simulink model "BrainihacksSampleDesignFinal"  (R2021b)
settings: Solver=VariableStepAuto  StartTime=0.0  StopTime=inf  RelTol=1e-3
undefined symbols (not defined in the file): fdesignblkfcn, gcbh, UN
libraries: dsparch4 x6, dspstat3 x2, simulink x2, slrealtimeiplib x1, UnicornLib x1
settings Model: Creator=Jos  LastModifiedBy=Jos

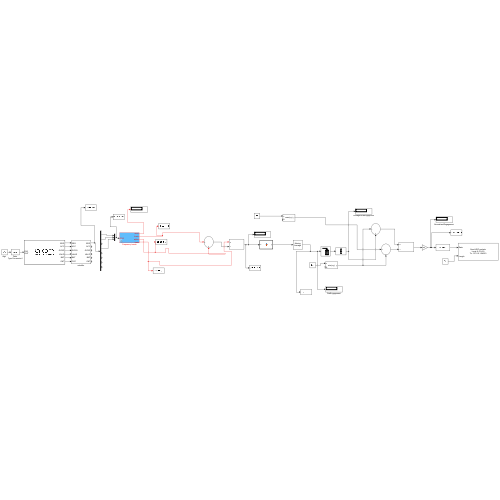
[thumbnail: Simulink's stored preview of the top-level diagram]
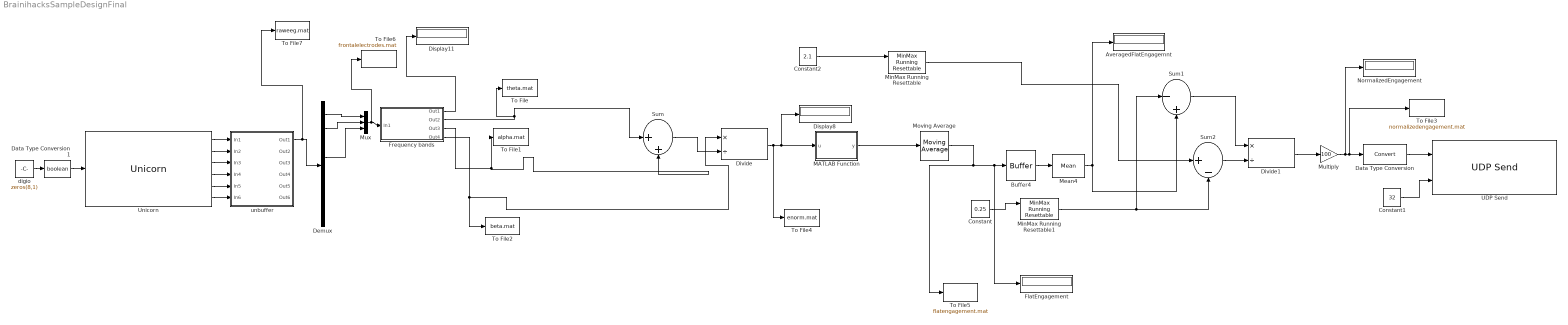
== system BrainihacksSampleDesignFinal ==
  AveragedFlatEngagemnt : Display
  Buffer4 : Buffer  N=128  OutputFrames=off
  Constant : Constant  Value=0.25
  Constant1 : Constant  Value=32
  Constant2 : Constant  Value=2.1
  Data Type Conversion1 : DataTypeConversion  OutDataTypeStr=boolean
  Data Type Conversion : DataTypeConversion
  Demux : Demux  Outputs=8
  Display11 : Display
  Display8 : Display
  Divide : Product  Inputs=*/
  Divide1 : Product  Inputs=*/
  FlatEngagement : Display
  Frequency bands : Subsystem  mask{windowLength=250, windowOverlap=240}
      mask prompts: windowLength "Window Length:"; windowOverlap "Window Overlap:"
      mask Display:
      | port_label('input',1,'EEG')
      | port_label('output',1,'delta')
      | port_label('output',2,'theta')
      | port_label('output',3,'alpha')
      | port_label('output',4,'beta')
  MATLAB Function : MATLAB Function  TreatAsAtomicUnit=on
  Mean4 : dspstat3/Mean  run=off  InputProcessing=Columns as channels (frame based)  reset_popup=None  directionMode=Each column  dimension=1  roiEnable=off  roiType=Rectangles  roiPortion=Entire ROI  roiOutput=Individual statistics for each ROI  roiFlag=off  roundingMode=Floor  overflowMode=off  outputDataTypeStr=Inherit: Same as accumulator  outputMin=[]  outputMax=[]  outputLastDataTypeStr=Inherit: Same as accumulator
  MinMax Running Resettable : simulink/Math Operations/MinMax Running Resettable  Function=max  vinit=0.0
  MinMax Running Resettable1 : simulink/Math Operations/MinMax Running Resettable  Function=min  vinit=0.0
  Moving Average : dspstat3/Moving Average  Method=Exponential weighting  ForgettingFactorPort=off  SpecifyWindowLength=on  WindowLength=4  ForgettingFactor=0.9  SimulateUsing=Code generation
  Multiply : Gain  Gain=100
  Mux : Mux  Inputs=3
  NormalizedEngagement : Display
  Sum : Sum  Inputs=|++
  Sum1 : Sum  Inputs=|-+
  Sum2 : Sum  Inputs=|+-
  To File : ToFile  Filename=theta.mat  SaveFormat=Timeseries
  To File1 : ToFile  Filename=alpha.mat  SaveFormat=Timeseries
  To File2 : ToFile  Filename=beta.mat  SaveFormat=Timeseries
  To File3 : ToFile  Filename=normalizedengagement.mat  SaveFormat=Timeseries
  To File4 : ToFile  Filename=enorm.mat  SaveFormat=Timeseries
  To File5 : ToFile  Filename=flatengagement.mat  SaveFormat=Timeseries
  To File6 : ToFile  Filename=frontalelectrodes.mat  SaveFormat=Timeseries
  To File7 : ToFile  Filename=raweeg.mat  SaveFormat=Timeseries
  UDP Send : slrealtimeiplib/UDP Send  useHostTargetConn=off  toAddress='127.0.0.1'  toPort=54320  sampleTime=-1
      settings: SourceProductBaseCode=XP
  Unicorn : UnicornLib/Unicorn  serial=UN-2019.05.55  old_serial=UN-2019.05.55  frame_length=1  input_source=Electrode
      settings: SourceProductName=Unicorn
  digio : Constant  Value=zeros(8,1)  SampleTime=-1
  "unbuffer " : Subsystem
      mask Display:
      | port_label('input',1,'EEG')
      | port_label('input',2,'ACC')
      | port_label('input',3,'GYRO')
      | port_label('input',4,'VALID')
      | port_label('input',5,'BAT')
      | port_label('input',6,'CNT')
      | port_label('output',1,'EEG')
      | port_label('output',2,'ACC')
      | port_label('output',3,'GYRO')
      | port_label('output',4,'VALID')
      | port_label('output',5,'BAT')
      | port_label('output',6,'CNT')
  wires:
  Unicorn/2 -> "unbuffer "/2(In2)
  Data Type Conversion1/1 -> Unicorn/1
  Unicorn/4 -> "unbuffer "/4(In4)
  Unicorn/5 -> "unbuffer "/5(In5)
  digio/1 -> Data Type Conversion1/1
  Unicorn/3 -> "unbuffer "/3(In3)
  Unicorn/6 -> "unbuffer "/6(In6)
  Unicorn/1 -> "unbuffer "/1(In1)
  Sum1/1 -> Divide1/1
  MinMax Running Resettable1/1 -> Sum1/1, Sum2/2
  Frequency bands/3(Out3) -> Sum/2, To File1/1
  Constant1/1 -> UDP Send/2
  Sum2/1 -> Divide1/2
  Sum/1 -> Divide/2
  MinMax Running Resettable/1 -> Sum2/1
  Data Type Conversion/1 -> UDP Send/1
  Frequency bands/4(Out4) -> Divide/1, To File2/1
  Constant/1 -> MinMax Running Resettable1/1
  Multiply/1 -> NormalizedEngagement/1, To File3/1, Data Type Conversion/1
  "unbuffer "/1(Out1) -> To File7/1, Demux/1
  Mux/1 -> To File6/1, Frequency bands/1(In1)
  Demux/1 -> Mux/1
  Demux/2 -> Mux/2
  Demux/4 -> Mux/3
  Divide1/1 -> Multiply/1
  Frequency bands/2(Out2) -> Sum/1, To File/1
  Buffer4/1 -> Mean4/1
  Mean4/1 -> Sum1/2, AveragedFlatEngagemnt/1
  Constant2/1 -> MinMax Running Resettable/1
  Moving Average/1 -> Buffer4/1, FlatEngagement/1, To File5/1
  Divide/1 -> Display8/1, MATLAB Function/1(u), To File4/1
  MATLAB Function/1(y) -> Moving Average/1
  Frequency bands/1(Out1) -> Display11/1

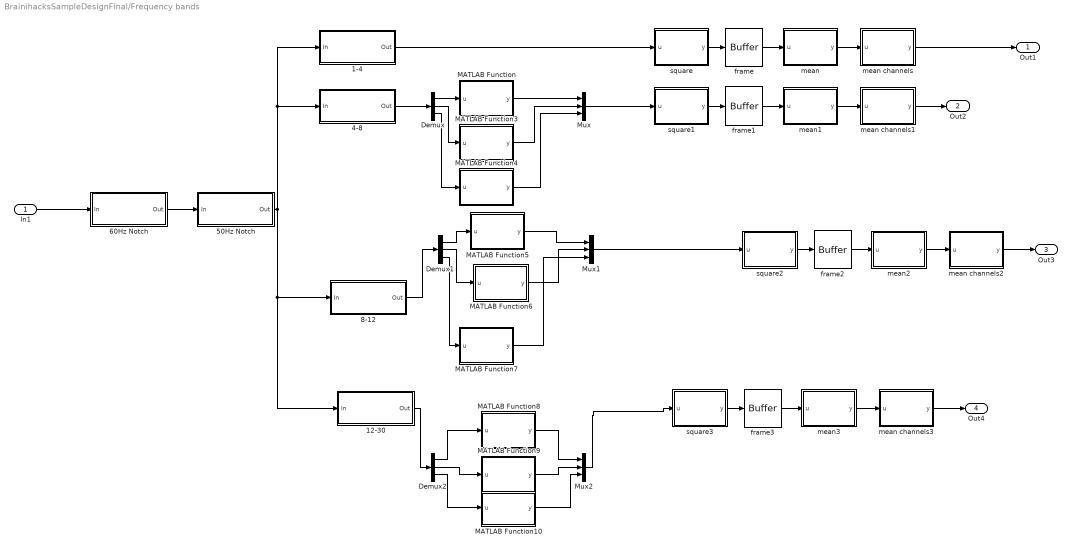
== system BrainihacksSampleDesignFinal/Frequency bands ==
  In1 : Inport
  1-4 : Subsystem  DialogController=fdesignblkfcn  InitFcn=fdesignblkfcn(gcbh, {'InitFcn'});  mask(Bandpass Filter){}
      mask help: Design a bandpass filter
      settings: CopyFcn=fdesignblkfcn(gcbh, {'CopyFcn'});
      mask Help: helpview(mapfilelocation('dsp'), 'dspbandpassfilter');
      mask Display: disp('Bandpass');
  12-30 : Subsystem  DialogController=fdesignblkfcn  InitFcn=fdesignblkfcn(gcbh, {'InitFcn'});  mask(Bandpass Filter){}
      mask help: Design a bandpass filter
      settings: CopyFcn=fdesignblkfcn(gcbh, {'CopyFcn'});
      mask Help: helpview(mapfilelocation('dsp'), 'dspbandpassfilter');
      mask Display: disp('Bandpass');
  4-8 : Subsystem  DialogController=fdesignblkfcn  InitFcn=fdesignblkfcn(gcbh, {'InitFcn'});  mask(Bandpass Filter){}
      mask help: Design a bandpass filter
      settings: CopyFcn=fdesignblkfcn(gcbh, {'CopyFcn'});
      mask Help: helpview(mapfilelocation('dsp'), 'dspbandpassfilter');
      mask Display: disp('Bandpass');
  50Hz Notch : Subsystem  DialogController=fdesignblkfcn  InitFcn=fdesignblkfcn(gcbh, {'InitFcn'});  mask(Bandstop Filter){}
      mask help: Design a bandstop filter
      settings: CopyFcn=fdesignblkfcn(gcbh, {'CopyFcn'});
      mask Help: helpview(mapfilelocation('dsp'), 'dspbandstopfilter');
      mask Display: disp('Bandstop');
  60Hz Notch : Subsystem  DialogController=fdesignblkfcn  InitFcn=fdesignblkfcn(gcbh, {'InitFcn'});  mask(Bandstop Filter){}
      mask help: Design a bandstop filter
      settings: CopyFcn=fdesignblkfcn(gcbh, {'CopyFcn'});
      mask Help: helpview(mapfilelocation('dsp'), 'dspbandstopfilter');
      mask Display: disp('Bandstop');
  8-12 : Subsystem  DialogController=fdesignblkfcn  InitFcn=fdesignblkfcn(gcbh, {'InitFcn'});  mask(Bandpass Filter){}
      mask help: Design a bandpass filter
      settings: CopyFcn=fdesignblkfcn(gcbh, {'CopyFcn'});
      mask Help: helpview(mapfilelocation('dsp'), 'dspbandpassfilter');
      mask Display: disp('Bandpass');
  Demux : Demux  Outputs=3
  Demux1 : Demux  Outputs=3
  Demux2 : Demux  Outputs=3
  MATLAB Function : MATLAB Function  TreatAsAtomicUnit=on
  MATLAB Function10 : MATLAB Function  TreatAsAtomicUnit=on
  MATLAB Function3 : MATLAB Function  TreatAsAtomicUnit=on
  MATLAB Function4 : MATLAB Function  TreatAsAtomicUnit=on
  MATLAB Function5 : MATLAB Function  TreatAsAtomicUnit=on
  MATLAB Function6 : MATLAB Function  TreatAsAtomicUnit=on
  MATLAB Function7 : MATLAB Function  TreatAsAtomicUnit=on
  MATLAB Function8 : MATLAB Function  TreatAsAtomicUnit=on
  MATLAB Function9 : MATLAB Function  TreatAsAtomicUnit=on
  Mux : Mux  Inputs=3
  Mux1 : Mux  Inputs=3
  Mux2 : Mux  Inputs=3
  frame{,1..3} (4 alike) : Buffer  N=windowLength  V=windowOverlap
  mean : MATLAB Function  TreatAsAtomicUnit=on
  mean channels : MATLAB Function  TreatAsAtomicUnit=on
  mean channels1 : MATLAB Function  TreatAsAtomicUnit=on
  mean channels2 : MATLAB Function  TreatAsAtomicUnit=on
  mean channels3 : MATLAB Function  TreatAsAtomicUnit=on
  mean1 : MATLAB Function  TreatAsAtomicUnit=on
  mean2 : MATLAB Function  TreatAsAtomicUnit=on
  mean3 : MATLAB Function  TreatAsAtomicUnit=on
  square : MATLAB Function  TreatAsAtomicUnit=on
  square1 : MATLAB Function  TreatAsAtomicUnit=on
  square2 : MATLAB Function  TreatAsAtomicUnit=on
  square3 : MATLAB Function  TreatAsAtomicUnit=on
  Out1 : Outport
  Out2 : Outport  Port=2
  Out3 : Outport  Port=3
  Out4 : Outport  Port=4
  wires:
  In1/1 -> 60Hz Notch/1(In)
  50Hz Notch/1(Out) -> 8-12/1(In), 12-30/1(In), 4-8/1(In), 1-4/1(In)
  60Hz Notch/1(Out) -> 50Hz Notch/1(In)
  square/1(y) -> frame/1
  mean/1(y) -> mean channels/1(u)
  frame/1 -> mean/1(u)
  square3/1(y) -> frame3/1
  frame3/1 -> mean3/1(u)
  mean3/1(y) -> mean channels3/1(u)
  frame1/1 -> mean1/1(u)
  mean1/1(y) -> mean channels1/1(u)
  square1/1(y) -> frame1/1
  mean2/1(y) -> mean channels2/1(u)
  square2/1(y) -> frame2/1
  frame2/1 -> mean2/1(u)
  mean channels3/1(y) -> Out4/1
  mean channels2/1(y) -> Out3/1
  mean channels1/1(y) -> Out2/1
  mean channels/1(y) -> Out1/1
  Mux2/1 -> square3/1(u)
  Mux1/1 -> square2/1(u)
  1-4/1(Out) -> square/1(u)
  4-8/1(Out) -> Demux/1
  Demux/1 -> MATLAB Function/1(u)
  Demux/2 -> MATLAB Function3/1(u)
  Demux/3 -> MATLAB Function4/1(u)
  MATLAB Function/1(y) -> Mux/1
  MATLAB Function3/1(y) -> Mux/2
  MATLAB Function4/1(y) -> Mux/3
  Mux/1 -> square1/1(u)
  Demux1/1 -> MATLAB Function5/1(u)
  MATLAB Function5/1(y) -> Mux1/1
  MATLAB Function6/1(y) -> Mux1/2
  MATLAB Function7/1(y) -> Mux1/3
  Demux1/2 -> MATLAB Function6/1(u)
  Demux1/3 -> MATLAB Function7/1(u)
  8-12/1(Out) -> Demux1/1
  Demux2/1 -> MATLAB Function8/1(u)
  Demux2/2 -> MATLAB Function9/1(u)
  Demux2/3 -> MATLAB Function10/1(u)
  MATLAB Function8/1(y) -> Mux2/1
  MATLAB Function9/1(y) -> Mux2/2
  MATLAB Function10/1(y) -> Mux2/3
  12-30/1(Out) -> Demux2/1

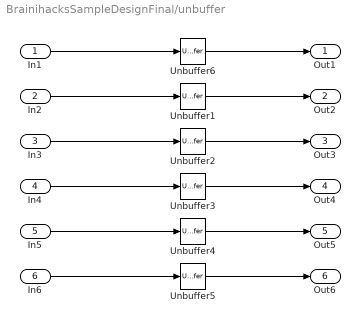
== system BrainihacksSampleDesignFinal/unbuffer  ==
  In1 : Inport
  In2 : Inport  Port=2
  In3 : Inport  Port=3
  In4 : Inport  Port=4
  In5 : Inport  Port=5
  In6 : Inport  Port=6
  Unbuffer{1..6} (6 alike) : Unbuffer
  Out1 : Outport
  Out2 : Outport  Port=2
  Out3 : Outport  Port=3
  Out4 : Outport  Port=4
  Out5 : Outport  Port=5
  Out6 : Outport  Port=6
  wires:
  In1/1 -> Unbuffer6/1
  In6/1 -> Unbuffer5/1
  In2/1 -> Unbuffer1/1
  In3/1 -> Unbuffer2/1
  In4/1 -> Unbuffer3/1
  In5/1 -> Unbuffer4/1
  Unbuffer4/1 -> Out5/1
  Unbuffer5/1 -> Out6/1
  Unbuffer3/1 -> Out4/1
  Unbuffer2/1 -> Out3/1
  Unbuffer1/1 -> Out2/1
  Unbuffer6/1 -> Out1/1

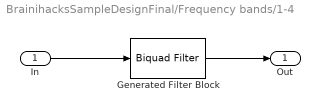
== system BrainihacksSampleDesignFinal/Frequency bands/1-4 ==
  In : Inport
  Generated Filter Block : dsparch4/Biquad Filter  Tag=BlockMethodSubSystem  FilterSource=Dialog parameters  CoeffSource=Specify via dialog  FilterObject=Hm_biquad  IIRFiltStruct=Direct form II  BiQuadCoeffs=[0.15421614382282306 0 -0.15421614382282306 1 -1.9591455332915735 0.96021687120286581;0.045953106150350399 0 -0.045953106150350399 1 -1.938666052126687 0.94767750927495009;0.048689091381584851 0 -0.048689091381584851 1 -1.9131195302980992 0.91652858121637504;0.008905390443523736 0 -0.008905390443523736 1 -1.9048500689711947 0.91042901788561015;0.0072890587489575177 0 -0.0072890587489575177 1 -1.9946197261392864 0.99525586386156895;0.03648759344543246 0 -0.03648759344543246 1 -1.9847418936203076 0.98542626556011315;0.13593808781804081 0 -0.13593808781804081 1 -1.9382239925127123 0.93996536435017564;0.17102469015765884 0 -0.17102469015765884 1 -1.9150503369448679 0.92256979274094753;0.013016622522025073 0 -0.013016622522025073 1 -1.9714532744309086 0.98136277878560862;2 0 -2 1 -1.9734938643446944 0.97429918172884178]  ScaleValues=[0.0010383082586855816;1;1;1;1;1;1;1;1;1;8.9140618887536736]  IC=0  ICnum=0  ICden=0  a0Flag=Warning  optimizeScaleValues=on  ScaleValueMode=Specify via input port (g)  roundingMode=Floor  overflowMode=off  scaleValueFracLength=14  denProdOutputFracLength=30  denAccumFracLength=30  secondMemoryFracLength=15
  Out : Outport
  wires:
  In/1 -> Generated Filter Block/1
  Generated Filter Block/1 -> Out/1

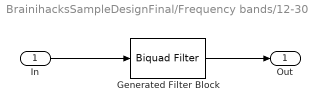
== system BrainihacksSampleDesignFinal/Frequency bands/12-30 ==
  In : Inport
  Generated Filter Block : dsparch4/Biquad Filter  Tag=BlockMethodSubSystem  FilterSource=Dialog parameters  CoeffSource=Specify via dialog  FilterObject=Hm_biquad  IIRFiltStruct=Direct form II  BiQuadCoeffs=[0.25062308717593751 0 -0.25062308717593751 1 -1.3148212076988803 0.75950452270759317;0.20862161434189525 0 -0.20862161434189525 1 -1.6037935286072298 0.72589040536938054;0.19851979389385729 0 -0.19851979389385729 1 -1.3911667358501223 0.60669985022096273;0.088137684162421806 0 -0.088137684162421806 1 -1.316886646759305 0.60531816515023407;0.24848271373823119 0 -0.24848271373823119 1 -1.8700123300550717 0.95920790693655777;0.17594128264449563 0 -0.17594128264449563 1 -1.3955906178302282 0.90907628614007652;0.2589480345611031 0 -0.2589480345611031 1 -1.2896771468564396 0.65708819345346747;0.28565593263291539 0 -0.28565593263291539 1 -1.4956371668923192 0.65420715584362399;0.13348297618292909 0 -0.13348297618292909 1 -1.7887919209725538 0.8806099427037436;1.5484038472870303 0 -1.5484038472870303 1 -1.701476495877744 0.80321292494565044]  ScaleValues=[0.15787933186786271;1;1;1;1;1;1;1;1;1;1]  IC=0  ICnum=0  ICden=0  a0Flag=Warning  optimizeScaleValues=on  ScaleValueMode=Specify via input port (g)  roundingMode=Floor  overflowMode=off  scaleValueFracLength=14  denProdOutputFracLength=30  denAccumFracLength=30  secondMemoryFracLength=15
  Out : Outport
  wires:
  In/1 -> Generated Filter Block/1
  Generated Filter Block/1 -> Out/1

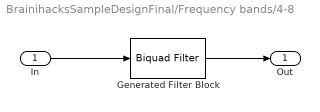
== system BrainihacksSampleDesignFinal/Frequency bands/4-8 ==
  In : Inport
  Generated Filter Block : dsparch4/Biquad Filter  Tag=BlockMethodSubSystem  FilterSource=Dialog parameters  CoeffSource=Specify via dialog  FilterObject=Hm_biquad  IIRFiltStruct=Direct form II  BiQuadCoeffs=[0.063242286603285194 0 -0.063242286603285194 1 -1.9057227294353984 0.94237189630698637;0.05033645981365821 0 -0.05033645981365821 1 -1.9140140114524609 0.92792511023439761;0.053006078153287083 0 -0.053006078153287083 1 -1.8739106619593258 0.90075619873998336;0.023565922726807367 0 -0.023565922726807367 1 -1.8784804701714481 0.90006654774644446;0.049652407322763166 0 -0.049652407322763166 1 -1.9793834245551323 0.98950211514928177;0.043821243540929505 0 -0.043821243540929505 1 -1.9397807008178365 0.9793665769679869;0.065946352755122908 0 -0.065946352755122908 1 -1.8829442008892903 0.9150980923191645;0.06855659790882572 0 -0.06855659790882572 1 -1.8934820031361492 0.91062981820568545;0.03757015493351671 0 -0.03757015493351671 1 -1.9580496612054441 0.96866699866189854;2 0 -2 1 -1.9361407076098807 0.94795535153308841]  ScaleValues=[0.011014898877795627;1;1;1;1;1;1;1;1;1;2.3254927592952472]  IC=0  ICnum=0  ICden=0  a0Flag=Warning  optimizeScaleValues=on  ScaleValueMode=Specify via input port (g)  roundingMode=Floor  overflowMode=off  scaleValueFracLength=14  denProdOutputFracLength=30  denAccumFracLength=30  secondMemoryFracLength=15
  Out : Outport
  wires:
  In/1 -> Generated Filter Block/1
  Generated Filter Block/1 -> Out/1

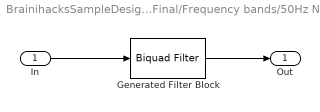
== system BrainihacksSampleDesignFinal/Frequency bands/50Hz Notch ==
  In : Inport
  Generated Filter Block : dsparch4/Biquad Filter  Tag=BlockMethodSubSystem  FilterSource=Dialog parameters  CoeffSource=Specify via dialog  FilterObject=Hm_biquad  IIRFiltStruct=Direct form II  BiQuadCoeffs=[2 -1.2376311593598059 1.9999999999999996 1 -0.58917542534408363 0.90420359373902093]  ScaleValues=[0.091083863875771748;5.226511899890804]  IC=0  ICnum=0  ICden=0  a0Flag=Warning  optimizeScaleValues=on  ScaleValueMode=Specify via input port (g)  roundingMode=Floor  overflowMode=off  scaleValueFracLength=14  denProdOutputFracLength=30  denAccumFracLength=30  secondMemoryFracLength=15
  Out : Outport
  wires:
  Generated Filter Block/1 -> Out/1
  In/1 -> Generated Filter Block/1

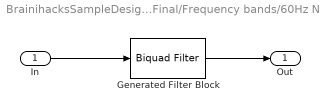
== system BrainihacksSampleDesignFinal/Frequency bands/60Hz Notch ==
  In : Inport
  Generated Filter Block : dsparch4/Biquad Filter  Tag=BlockMethodSubSystem  FilterSource=Dialog parameters  CoeffSource=Specify via dialog  FilterObject=Hm_biquad  IIRFiltStruct=Direct form II  BiQuadCoeffs=[1.9999999999999998 -0.25147970790103907 2 1 -0.11971714088439944 0.90420359373902071]  ScaleValues=[0.095607010933771011;4.9792467496397919]  IC=0  ICnum=0  ICden=0  a0Flag=Warning  optimizeScaleValues=on  ScaleValueMode=Specify via input port (g)  roundingMode=Floor  overflowMode=off  scaleValueFracLength=14  denProdOutputFracLength=30  denAccumFracLength=30  secondMemoryFracLength=15
  Out : Outport
  wires:
  Generated Filter Block/1 -> Out/1
  In/1 -> Generated Filter Block/1

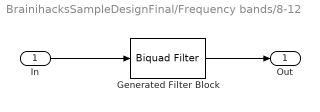
== system BrainihacksSampleDesignFinal/Frequency bands/8-12 ==
  In : Inport
  Generated Filter Block : dsparch4/Biquad Filter  Tag=BlockMethodSubSystem  FilterSource=Dialog parameters  CoeffSource=Specify via dialog  FilterObject=Hm_biquad  IIRFiltStruct=Direct form II  BiQuadCoeffs=[0.086508931071228451 0 -0.086508931071228451 1 -1.8969516123540997 0.94080090381668036;0.054164091257831087 0 -0.054164091257831087 1 -1.8446099162440039 0.92205707952922966;0.04893737073757258 0 -0.04893737073757258 1 -1.8373112193826748 0.90672178009865512;0.018925317300337391 0 -0.018925317300337391 1 -1.841166803183204 0.90245599667915;0.087704899838196362 0 -0.087704899838196362 1 -1.9471939371001552 0.9874201547495447;0.059365063980243639 0 -0.059365063980243639 1 -1.892415306235564 0.98143155652128711;0.053411232433961571 0 -0.053411232433961571 1 -1.8737225939070978 0.92182002611558977;0.01967405559358212 0 -0.01967405559358212 1 -1.8542288257633226 0.90821872729908426;0.1069534166772903 0 -0.1069534166772903 1 -1.9218814308059495 0.96313134833879099;2 0 -2 1 -1.8634604713625618 0.94778823053935468]  ScaleValues=[0.012387569116855223;1;1;1;1;1;1;1;1;1;1.1967009601971133]  IC=0  ICnum=0  ICden=0  a0Flag=Warning  optimizeScaleValues=on  ScaleValueMode=Specify via input port (g)  roundingMode=Floor  overflowMode=off  scaleValueFracLength=14  denProdOutputFracLength=30  denAccumFracLength=30  secondMemoryFracLength=15
  Out : Outport
  wires:
  In/1 -> Generated Filter Block/1
  Generated Filter Block/1 -> Out/1

== matlab function BrainihacksSampleDesignFinal/Frequency bands/MATLAB Function3 ==
  data: u input; y output
function y = fcn(u)
%if u < 20
%    u = 20;
if u > 100
    u = 100;
end

y = u;

== matlab function BrainihacksSampleDesignFinal/Frequency bands/MATLAB Function4 ==
  data: u input; y output
function y = fcn(u)
%if u < 20
%    u = 20;
if u > 100
    u = 100;
end

y = u;

== matlab function BrainihacksSampleDesignFinal/Frequency bands/MATLAB Function5 ==
  data: u input; y output
function y = fcn(u)
%if u < 20
%    u = 20;
if u >60
    u = 60;
end
y = u;

== matlab function BrainihacksSampleDesignFinal/Frequency bands/MATLAB Function6 ==
  data: u input; y output
function y = fcn(u)
%if u < 20
%    u = 20;
if u >60
    u = 60;
end
y = u;

== matlab function BrainihacksSampleDesignFinal/Frequency bands/MATLAB Function7 ==
  data: u input; y output
function y = fcn(u)
%if u < 20
%    u = 20;
if u >60
    u = 60;
end
y = u;

== matlab function BrainihacksSampleDesignFinal/Frequency bands/square ==
  data: u input; y output
function y = fcn(u)
for i=1:length(u)
    u(i)=u(i)*u(i);
end
y = u;

== matlab function BrainihacksSampleDesignFinal/Frequency bands/MATLAB Function8 ==
  data: u input; y output
function y = fcn(u)
%if u < 2
%    u = 2;
if u > 20
    u = 20;
end
y = u;

== matlab function BrainihacksSampleDesignFinal/Frequency bands/MATLAB Function9 ==
  data: u input; y output
function y = fcn(u)
%if u < 2
%    u = 2;
if u > 20
    u = 20;
end
y = u;

== matlab function BrainihacksSampleDesignFinal/Frequency bands/MATLAB Function10 ==
  data: u input; y output
function y = fcn(u)
%if u < 2
%    u = 2;
if u > 20
    u = 20;
end
y = u;

== matlab function BrainihacksSampleDesignFinal/Frequency bands/mean channels ==
  data: u input; y output
function y = fcn(u)
y=mean(u);

== matlab function BrainihacksSampleDesignFinal/Frequency bands/mean channels1 ==
  data: u input; y output
function y = fcn(u)
y=mean(u);

== matlab function BrainihacksSampleDesignFinal/Frequency bands/mean1 ==
  data: u input; y output
function y = fcn(u)
[~,c]=size(u);
x = zeros(c,1);
for i=1:c
    x(i)=mean(u(:,i));
end
y=x;

== matlab function BrainihacksSampleDesignFinal/Frequency bands/square1 ==
  data: u input; y output
function y = fcn(u)
for i=1:length(u)
    u(i)=u(i)*u(i);
end
y = u;

== matlab function BrainihacksSampleDesignFinal/Frequency bands/mean channels2 ==
  data: u input; y output
function y = fcn(u)
y=mean(u);

== matlab function BrainihacksSampleDesignFinal/Frequency bands/mean2 ==
  data: u input; y output
function y = fcn(u)
[~,c]=size(u);
x = zeros(c,1);
for i=1:c
    x(i)=mean(u(:,i));
end
y=x;

== matlab function BrainihacksSampleDesignFinal/Frequency bands/square2 ==
  data: u input; y output
function y = fcn(u)
for i=1:length(u)
    u(i)=u(i)*u(i);
end
y = u;

== matlab function BrainihacksSampleDesignFinal/Frequency bands/mean ==
  data: u input; y output
function y = fcn(u)
[~,c]=size(u);
x = zeros(c,1);
for i=1:c
    x(i)=mean(u(:,i));
end
y=x;

== matlab function BrainihacksSampleDesignFinal/Frequency bands/mean channels3 ==
  data: u input; y output
function y = fcn(u)
y=mean(u);

== matlab function BrainihacksSampleDesignFinal/Frequency bands/mean3 ==
  data: u input; y output
function y = fcn(u)
[~,c]=size(u);
x = zeros(c,1);
for i=1:c
    x(i)=mean(u(:,i));
end
y=x;

== matlab function BrainihacksSampleDesignFinal/Frequency bands/square3 ==
  data: u input; y output
function y = fcn(u)
for i=1:length(u)
    u(i)=u(i)*u(i);
end
y = u;

== matlab function BrainihacksSampleDesignFinal/MATLAB Function ==
  data: u input; y output
function y = fcn(u)
if (isnan(u))
    u = 1;
end
y = u;

== matlab function BrainihacksSampleDesignFinal/Frequency bands/MATLAB Function ==
  data: u input; y output
function y = fcn(u)
%if u < 20
 %   u = 20;
if u > 100
    u = 100;
end

y = u;
